simulink model "AariaJoystickR2017a"  (R2017a)
settings: Solver=VariableStepAuto  StartTime=0.0  StopTime=inf  FixedStep=0.1  RelTol=1e-3  EnableMultiTasking=on
model workspace (MATLAB code in the model file):
  | my_a =1;
undefined symbols (not defined in the file or in its folder): AARIAENV, AARIAMAN, AARIASEN, Camera, sensor, Source_TS, X, Y, Z
libraries: sm_lib x723, nesl_utility x640, dspmathops x314, simulink x168, vrlib x2, powerlib_meascontrol x1, aerolibanimutils x1, aerolibutil x1
(part 16 of 26)

== system AariaJoystickR2017a/Joint2/JointVSS/PrismaticTorque/IMU Sensors/Sensor Module1 ==
  Gain : Gain  Gain=1/AARIAENV.Min_TS
  Gain1 : Gain  Gain=1/AARIAENV.Min_TS^2
  Gain3 : Gain  Gain=AARIAENV.gravity  Multiplication=Matrix(K*u)
  Mux : Mux  Inputs=3
  Mux1 : Mux  Inputs=3
  Mux2 : Mux  Inputs=3
  PS-Simulink Converter{5..11} (7 alike) : nesl_utility/PS-Simulink Converter  PhysicalDomain=network_engine_domain  SubClassName=ps_output  LeftPortType=input  RightPortType=output  PseudoPeriodic=off  Frequencies=[]  Unit=1  AffineConversion=off
  PS-Simulink Converter2 : nesl_utility/PS-Simulink Converter  PhysicalDomain=network_engine_domain  SubClassName=ps_output  LeftPortType=input  RightPortType=output  PseudoPeriodic=off  Frequencies=[]  Unit=rad/s  AffineConversion=off
  PS-Simulink Converter3 : nesl_utility/PS-Simulink Converter  PhysicalDomain=network_engine_domain  SubClassName=ps_output  LeftPortType=input  RightPortType=output  PseudoPeriodic=off  Frequencies=[]  Unit=rad/s  AffineConversion=off
  PS-Simulink Converter4 : nesl_utility/PS-Simulink Converter  PhysicalDomain=network_engine_domain  SubClassName=ps_output  LeftPortType=input  RightPortType=output  PseudoPeriodic=off  Frequencies=[]  Unit=rad/s  AffineConversion=off
  Sensor Place : sm_lib/Frames and Transforms/Rigid Transform  TranslationMethod=Cartesian  TranslationStandardOffset=0  TranslationLengthUnit=m  TranslationStandardAxis=+Z  TranslationCartesianOffset=AARIAMAN.L(nL).S(nS).pose_p  TranslationROffset=0  TranslationROffsetUnits=m  TranslationZOffset=0  TranslationZOffsetUnits=m  TranslationThetaOffset=0  TranslationThetaOffsetUnits=deg  RotationMethod=RotationMatrix  RotationAngleUnits=deg  RotationStandardAxis=+Z  RotationAngle=0.0  RotationArbitraryAxis=[0 0 1]  FollAlignAxisA=+X  BaseAlignAxisA=+Y  FollAlignAxisB=+Y  BaseAlignAxisB=+Z  RotationSequenceAxes=FollowerAxes  RotationSequence=XYX  RotationSequenceAngles=[0 0 0]  RotationSequenceAnglesUnits=deg  RotationMatrix=AARIAMAN.L(nL).S(nS).pose_r
  Sum : Sum  Inputs=|++
  Sum1 : Sum  Inputs=|++
  Sum2 : Sum  Inputs=++|
  Transform Sensor : sm_lib/Frames and Transforms/Transform Sensor  MeasurementFrame=Follower  SenseAngle=off  SenseAxis=off  SenseAngle1=off  SenseAngle2=off  SenseAngle3=off  SenseQ=off  SenseR=on  SenseOmegaX=on  SenseOmegaY=on  SenseOmegaZ=on  SenseOmega1=off  SenseOmega2=off  SenseOmega3=off  SenseQDot=off  SenseRDot=off  SenseAlphaX=off  SenseAlphaY=off  SenseAlphaZ=off  SenseAlpha1=off  SenseAlpha2=off  SenseAlpha3=off  SenseQDDot=off  SenseRDDot=off  SenseX=on  SenseY=on  SenseZ=on  SenseRad=off  SenseAzim=off  SenseDist=off  SenseInc=off  SenseXDot=off  SenseYDot=off  SenseZDot=off  SenseRadDot=off  SenseAzimDot=off  SenseDistDot=off  SenseIncDot=off  SenseXDDot=on  SenseYDDot=on  SenseZDDot=on  SenseRadDDot=off  SenseAzimDDot=off  SenseDistDDot=off  SenseIncDDot=off
  a_noise : Subsystem
  coord_sens : sm_lib/Body Elements/Graphic  GraphicType=Marker  MarkerShape=Frame  MarkerSize=AARIAMAN.vis.coord_sizeS  GraphicVisPropType=SimpleVisualProperties  GraphicDiffuseColor=AARIAMAN.vis.col_s  GraphicSpecularColor=[0.5 0.5 0.5 1.0]  GraphicAmbientColor=[0.15 0.15 0.15 1.0]  GraphicEmissiveColor=[0.0 0.0 0.0 1.0]  GraphicShininess=75  GraphicOpacity=AARIAMAN.vis.opacity_s
      settings: SourceProductName=Simscape Multibody
  omega_noise : Subsystem
  Body Frame : PMIOPort  Port=1  Side=Left
  Reference Frame : PMIOPort  Port=2  Side=Left
  Out5 : Outport
  Out4 : Outport  Port=2
  Out2 : Outport  Port=3
  Out3 : Outport  Port=4
  wires:
  Gain1/1 -> Sum/1
  Gain/1 -> Sum2/2
  a_noise/1(noise) -> Sum1/2
  omega_noise/1(noise) -> Sum2/1
  Gain3/1 -> Sum/2  "a_measured"
  Sum1/1 -> Out4/1  "a_measured"
  PS-Simulink Converter10/1 -> Mux2/2
  Mux1/1 -> Out2/1  "P_actual"
  PS-Simulink Converter11/1 -> Mux2/3
  PS-Simulink Converter9/1 -> Mux2/1
  PS-Simulink Converter3/1 -> Mux/2
  PS-Simulink Converter2/1 -> Mux/1
  PS-Simulink Converter4/1 -> Mux/3
  Mux/1 -> Gain/1
  PS-Simulink Converter6/1 -> Mux1/2
  PS-Simulink Converter5/1 -> Mux1/1
  PS-Simulink Converter7/1 -> Mux1/3
  Mux2/1 -> Gain1/1
  PS-Simulink Converter8/1 -> Out3/1, Gain3/1  "R_actual"
  Sum/1 -> Sum1/1
  Sum2/1 -> Out5/1  "omega_measured"
  connections:
  Sensor Place/RConn1 -- coord_sens/RConn1 -- Transform Sensor/RConn1
  Transform Sensor/RConn11 -- PS-Simulink Converter11/LConn1
  Sensor Place/LConn1 -- Body Frame/RConn1
  Transform Sensor/RConn3 -- PS-Simulink Converter2/LConn1
  Transform Sensor/RConn9 -- PS-Simulink Converter9/LConn1
  Transform Sensor/RConn4 -- PS-Simulink Converter3/LConn1
  Transform Sensor/LConn1 -- Reference Frame/RConn1
  Transform Sensor/RConn5 -- PS-Simulink Converter4/LConn1
  Transform Sensor/RConn10 -- PS-Simulink Converter10/LConn1
  Transform Sensor/RConn6 -- PS-Simulink Converter5/LConn1
  PS-Simulink Converter8/LConn1 -- Transform Sensor/RConn2
  Transform Sensor/RConn8 -- PS-Simulink Converter7/LConn1
  Transform Sensor/RConn7 -- PS-Simulink Converter6/LConn1

== system AariaJoystickR2017a/Joint2/JointVSS/PrismaticTorque/IMU Sensors/Sensor Module2 ==
  Gain : Gain  Gain=1/AARIAENV.Min_TS
  Gain1 : Gain  Gain=1/AARIAENV.Min_TS^2
  Gain3 : Gain  Gain=AARIAENV.gravity  Multiplication=Matrix(K*u)
  Mux : Mux  Inputs=3
  Mux1 : Mux  Inputs=3
  Mux2 : Mux  Inputs=3
  PS-Simulink Converter{5..11} (7 alike) : nesl_utility/PS-Simulink Converter  PhysicalDomain=network_engine_domain  SubClassName=ps_output  LeftPortType=input  RightPortType=output  PseudoPeriodic=off  Frequencies=[]  Unit=1  AffineConversion=off
  PS-Simulink Converter2 : nesl_utility/PS-Simulink Converter  PhysicalDomain=network_engine_domain  SubClassName=ps_output  LeftPortType=input  RightPortType=output  PseudoPeriodic=off  Frequencies=[]  Unit=rad/s  AffineConversion=off
  PS-Simulink Converter3 : nesl_utility/PS-Simulink Converter  PhysicalDomain=network_engine_domain  SubClassName=ps_output  LeftPortType=input  RightPortType=output  PseudoPeriodic=off  Frequencies=[]  Unit=rad/s  AffineConversion=off
  PS-Simulink Converter4 : nesl_utility/PS-Simulink Converter  PhysicalDomain=network_engine_domain  SubClassName=ps_output  LeftPortType=input  RightPortType=output  PseudoPeriodic=off  Frequencies=[]  Unit=rad/s  AffineConversion=off
  Sensor Place : sm_lib/Frames and Transforms/Rigid Transform  TranslationMethod=Cartesian  TranslationStandardOffset=0  TranslationLengthUnit=m  TranslationStandardAxis=+Z  TranslationCartesianOffset=AARIAMAN.L(nL).S(nS).pose_p  TranslationROffset=0  TranslationROffsetUnits=m  TranslationZOffset=0  TranslationZOffsetUnits=m  TranslationThetaOffset=0  TranslationThetaOffsetUnits=deg  RotationMethod=RotationMatrix  RotationAngleUnits=deg  RotationStandardAxis=+Z  RotationAngle=0.0  RotationArbitraryAxis=[0 0 1]  FollAlignAxisA=+X  BaseAlignAxisA=+Y  FollAlignAxisB=+Y  BaseAlignAxisB=+Z  RotationSequenceAxes=FollowerAxes  RotationSequence=XYX  RotationSequenceAngles=[0 0 0]  RotationSequenceAnglesUnits=deg  RotationMatrix=AARIAMAN.L(nL).S(nS).pose_r
  Sum : Sum  Inputs=|++
  Sum1 : Sum  Inputs=|++
  Sum2 : Sum  Inputs=++|
  Transform Sensor : sm_lib/Frames and Transforms/Transform Sensor  MeasurementFrame=Follower  SenseAngle=off  SenseAxis=off  SenseAngle1=off  SenseAngle2=off  SenseAngle3=off  SenseQ=off  SenseR=on  SenseOmegaX=on  SenseOmegaY=on  SenseOmegaZ=on  SenseOmega1=off  SenseOmega2=off  SenseOmega3=off  SenseQDot=off  SenseRDot=off  SenseAlphaX=off  SenseAlphaY=off  SenseAlphaZ=off  SenseAlpha1=off  SenseAlpha2=off  SenseAlpha3=off  SenseQDDot=off  SenseRDDot=off  SenseX=on  SenseY=on  SenseZ=on  SenseRad=off  SenseAzim=off  SenseDist=off  SenseInc=off  SenseXDot=off  SenseYDot=off  SenseZDot=off  SenseRadDot=off  SenseAzimDot=off  SenseDistDot=off  SenseIncDot=off  SenseXDDot=on  SenseYDDot=on  SenseZDDot=on  SenseRadDDot=off  SenseAzimDDot=off  SenseDistDDot=off  SenseIncDDot=off
  a_noise : Subsystem
  coord_sens : sm_lib/Body Elements/Graphic  GraphicType=Marker  MarkerShape=Frame  MarkerSize=AARIAMAN.vis.coord_sizeS  GraphicVisPropType=SimpleVisualProperties  GraphicDiffuseColor=AARIAMAN.vis.col_s  GraphicSpecularColor=[0.5 0.5 0.5 1.0]  GraphicAmbientColor=[0.15 0.15 0.15 1.0]  GraphicEmissiveColor=[0.0 0.0 0.0 1.0]  GraphicShininess=75  GraphicOpacity=AARIAMAN.vis.opacity_s
      settings: SourceProductName=Simscape Multibody
  omega_noise : Subsystem
  Body Frame : PMIOPort  Port=1  Side=Left
  Reference Frame : PMIOPort  Port=2  Side=Left
  Out5 : Outport
  Out4 : Outport  Port=2
  Out2 : Outport  Port=3
  Out3 : Outport  Port=4
  wires:
  Gain1/1 -> Sum/1
  Gain/1 -> Sum2/2
  a_noise/1(noise) -> Sum1/2
  omega_noise/1(noise) -> Sum2/1
  Gain3/1 -> Sum/2  "a_measured"
  Sum1/1 -> Out4/1  "a_measured"
  PS-Simulink Converter10/1 -> Mux2/2
  Mux1/1 -> Out2/1  "P_actual"
  PS-Simulink Converter11/1 -> Mux2/3
  PS-Simulink Converter9/1 -> Mux2/1
  PS-Simulink Converter3/1 -> Mux/2
  PS-Simulink Converter2/1 -> Mux/1
  PS-Simulink Converter4/1 -> Mux/3
  Mux/1 -> Gain/1
  PS-Simulink Converter6/1 -> Mux1/2
  PS-Simulink Converter5/1 -> Mux1/1
  PS-Simulink Converter7/1 -> Mux1/3
  Mux2/1 -> Gain1/1
  PS-Simulink Converter8/1 -> Out3/1, Gain3/1  "R_actual"
  Sum/1 -> Sum1/1
  Sum2/1 -> Out5/1  "omega_measured"
  connections:
  Sensor Place/RConn1 -- coord_sens/RConn1 -- Transform Sensor/RConn1
  Transform Sensor/RConn11 -- PS-Simulink Converter11/LConn1
  Sensor Place/LConn1 -- Body Frame/RConn1
  Transform Sensor/RConn3 -- PS-Simulink Converter2/LConn1
  Transform Sensor/RConn9 -- PS-Simulink Converter9/LConn1
  Transform Sensor/RConn4 -- PS-Simulink Converter3/LConn1
  Transform Sensor/LConn1 -- Reference Frame/RConn1
  Transform Sensor/RConn5 -- PS-Simulink Converter4/LConn1
  Transform Sensor/RConn10 -- PS-Simulink Converter10/LConn1
  Transform Sensor/RConn6 -- PS-Simulink Converter5/LConn1
  PS-Simulink Converter8/LConn1 -- Transform Sensor/RConn2
  Transform Sensor/RConn8 -- PS-Simulink Converter7/LConn1
  Transform Sensor/RConn7 -- PS-Simulink Converter6/LConn1

== system AariaJoystickR2017a/Joint2/JointVSS/RevoluteMotion/IMU Sensors/Sensor Module1 ==
  Gain : Gain  Gain=1/AARIAENV.Min_TS
  Gain1 : Gain  Gain=1/AARIAENV.Min_TS^2
  Gain3 : Gain  Gain=AARIAENV.gravity  Multiplication=Matrix(K*u)
  Mux : Mux  Inputs=3
  Mux1 : Mux  Inputs=3
  Mux2 : Mux  Inputs=3
  PS-Simulink Converter{5..11} (7 alike) : nesl_utility/PS-Simulink Converter  PhysicalDomain=network_engine_domain  SubClassName=ps_output  LeftPortType=input  RightPortType=output  PseudoPeriodic=off  Frequencies=[]  Unit=1  AffineConversion=off
  PS-Simulink Converter2 : nesl_utility/PS-Simulink Converter  PhysicalDomain=network_engine_domain  SubClassName=ps_output  LeftPortType=input  RightPortType=output  PseudoPeriodic=off  Frequencies=[]  Unit=rad/s  AffineConversion=off
  PS-Simulink Converter3 : nesl_utility/PS-Simulink Converter  PhysicalDomain=network_engine_domain  SubClassName=ps_output  LeftPortType=input  RightPortType=output  PseudoPeriodic=off  Frequencies=[]  Unit=rad/s  AffineConversion=off
  PS-Simulink Converter4 : nesl_utility/PS-Simulink Converter  PhysicalDomain=network_engine_domain  SubClassName=ps_output  LeftPortType=input  RightPortType=output  PseudoPeriodic=off  Frequencies=[]  Unit=rad/s  AffineConversion=off
  Sensor Place : sm_lib/Frames and Transforms/Rigid Transform  TranslationMethod=Cartesian  TranslationStandardOffset=0  TranslationLengthUnit=m  TranslationStandardAxis=+Z  TranslationCartesianOffset=AARIAMAN.L(nL).S(nS).pose_p  TranslationROffset=0  TranslationROffsetUnits=m  TranslationZOffset=0  TranslationZOffsetUnits=m  TranslationThetaOffset=0  TranslationThetaOffsetUnits=deg  RotationMethod=RotationMatrix  RotationAngleUnits=deg  RotationStandardAxis=+Z  RotationAngle=0.0  RotationArbitraryAxis=[0 0 1]  FollAlignAxisA=+X  BaseAlignAxisA=+Y  FollAlignAxisB=+Y  BaseAlignAxisB=+Z  RotationSequenceAxes=FollowerAxes  RotationSequence=XYX  RotationSequenceAngles=[0 0 0]  RotationSequenceAnglesUnits=deg  RotationMatrix=AARIAMAN.L(nL).S(nS).pose_r
  Sum : Sum  Inputs=|++
  Sum1 : Sum  Inputs=|++
  Sum2 : Sum  Inputs=++|
  Transform Sensor : sm_lib/Frames and Transforms/Transform Sensor  MeasurementFrame=Follower  SenseAngle=off  SenseAxis=off  SenseAngle1=off  SenseAngle2=off  SenseAngle3=off  SenseQ=off  SenseR=on  SenseOmegaX=on  SenseOmegaY=on  SenseOmegaZ=on  SenseOmega1=off  SenseOmega2=off  SenseOmega3=off  SenseQDot=off  SenseRDot=off  SenseAlphaX=off  SenseAlphaY=off  SenseAlphaZ=off  SenseAlpha1=off  SenseAlpha2=off  SenseAlpha3=off  SenseQDDot=off  SenseRDDot=off  SenseX=on  SenseY=on  SenseZ=on  SenseRad=off  SenseAzim=off  SenseDist=off  SenseInc=off  SenseXDot=off  SenseYDot=off  SenseZDot=off  SenseRadDot=off  SenseAzimDot=off  SenseDistDot=off  SenseIncDot=off  SenseXDDot=on  SenseYDDot=on  SenseZDDot=on  SenseRadDDot=off  SenseAzimDDot=off  SenseDistDDot=off  SenseIncDDot=off
  a_noise : Subsystem
  coord_sens : sm_lib/Body Elements/Graphic  GraphicType=Marker  MarkerShape=Frame  MarkerSize=AARIAMAN.vis.coord_sizeS  GraphicVisPropType=SimpleVisualProperties  GraphicDiffuseColor=AARIAMAN.vis.col_s  GraphicSpecularColor=[0.5 0.5 0.5 1.0]  GraphicAmbientColor=[0.15 0.15 0.15 1.0]  GraphicEmissiveColor=[0.0 0.0 0.0 1.0]  GraphicShininess=75  GraphicOpacity=AARIAMAN.vis.opacity_s
      settings: SourceProductName=Simscape Multibody
  omega_noise : Subsystem
  Body Frame : PMIOPort  Port=1  Side=Left
  Reference Frame : PMIOPort  Port=2  Side=Left
  Out5 : Outport
  Out4 : Outport  Port=2
  Out2 : Outport  Port=3
  Out3 : Outport  Port=4
  wires:
  Gain1/1 -> Sum/1
  Gain/1 -> Sum2/2
  a_noise/1(noise) -> Sum1/2
  omega_noise/1(noise) -> Sum2/1
  Gain3/1 -> Sum/2  "a_measured"
  Sum1/1 -> Out4/1  "a_measured"
  PS-Simulink Converter10/1 -> Mux2/2
  Mux1/1 -> Out2/1  "P_actual"
  PS-Simulink Converter11/1 -> Mux2/3
  PS-Simulink Converter9/1 -> Mux2/1
  PS-Simulink Converter3/1 -> Mux/2
  PS-Simulink Converter2/1 -> Mux/1
  PS-Simulink Converter4/1 -> Mux/3
  Mux/1 -> Gain/1
  PS-Simulink Converter6/1 -> Mux1/2
  PS-Simulink Converter5/1 -> Mux1/1
  PS-Simulink Converter7/1 -> Mux1/3
  Mux2/1 -> Gain1/1
  PS-Simulink Converter8/1 -> Out3/1, Gain3/1  "R_actual"
  Sum/1 -> Sum1/1
  Sum2/1 -> Out5/1  "omega_measured"
  connections:
  Sensor Place/RConn1 -- coord_sens/RConn1 -- Transform Sensor/RConn1
  Transform Sensor/RConn11 -- PS-Simulink Converter11/LConn1
  Sensor Place/LConn1 -- Body Frame/RConn1
  Transform Sensor/RConn3 -- PS-Simulink Converter2/LConn1
  Transform Sensor/RConn9 -- PS-Simulink Converter9/LConn1
  Transform Sensor/RConn4 -- PS-Simulink Converter3/LConn1
  Transform Sensor/LConn1 -- Reference Frame/RConn1
  Transform Sensor/RConn5 -- PS-Simulink Converter4/LConn1
  Transform Sensor/RConn10 -- PS-Simulink Converter10/LConn1
  Transform Sensor/RConn6 -- PS-Simulink Converter5/LConn1
  PS-Simulink Converter8/LConn1 -- Transform Sensor/RConn2
  Transform Sensor/RConn8 -- PS-Simulink Converter7/LConn1
  Transform Sensor/RConn7 -- PS-Simulink Converter6/LConn1

== system AariaJoystickR2017a/Joint2/JointVSS/RevoluteMotion/IMU Sensors/Sensor Module2 ==
  Gain : Gain  Gain=1/AARIAENV.Min_TS
  Gain1 : Gain  Gain=1/AARIAENV.Min_TS^2
  Gain3 : Gain  Gain=AARIAENV.gravity  Multiplication=Matrix(K*u)
  Mux : Mux  Inputs=3
  Mux1 : Mux  Inputs=3
  Mux2 : Mux  Inputs=3
  PS-Simulink Converter{5..11} (7 alike) : nesl_utility/PS-Simulink Converter  PhysicalDomain=network_engine_domain  SubClassName=ps_output  LeftPortType=input  RightPortType=output  PseudoPeriodic=off  Frequencies=[]  Unit=1  AffineConversion=off
  PS-Simulink Converter2 : nesl_utility/PS-Simulink Converter  PhysicalDomain=network_engine_domain  SubClassName=ps_output  LeftPortType=input  RightPortType=output  PseudoPeriodic=off  Frequencies=[]  Unit=rad/s  AffineConversion=off
  PS-Simulink Converter3 : nesl_utility/PS-Simulink Converter  PhysicalDomain=network_engine_domain  SubClassName=ps_output  LeftPortType=input  RightPortType=output  PseudoPeriodic=off  Frequencies=[]  Unit=rad/s  AffineConversion=off
  PS-Simulink Converter4 : nesl_utility/PS-Simulink Converter  PhysicalDomain=network_engine_domain  SubClassName=ps_output  LeftPortType=input  RightPortType=output  PseudoPeriodic=off  Frequencies=[]  Unit=rad/s  AffineConversion=off
  Sensor Place : sm_lib/Frames and Transforms/Rigid Transform  TranslationMethod=Cartesian  TranslationStandardOffset=0  TranslationLengthUnit=m  TranslationStandardAxis=+Z  TranslationCartesianOffset=AARIAMAN.L(nL).S(nS).pose_p  TranslationROffset=0  TranslationROffsetUnits=m  TranslationZOffset=0  TranslationZOffsetUnits=m  TranslationThetaOffset=0  TranslationThetaOffsetUnits=deg  RotationMethod=RotationMatrix  RotationAngleUnits=deg  RotationStandardAxis=+Z  RotationAngle=0.0  RotationArbitraryAxis=[0 0 1]  FollAlignAxisA=+X  BaseAlignAxisA=+Y  FollAlignAxisB=+Y  BaseAlignAxisB=+Z  RotationSequenceAxes=FollowerAxes  RotationSequence=XYX  RotationSequenceAngles=[0 0 0]  RotationSequenceAnglesUnits=deg  RotationMatrix=AARIAMAN.L(nL).S(nS).pose_r
  Sum : Sum  Inputs=|++
  Sum1 : Sum  Inputs=|++
  Sum2 : Sum  Inputs=++|
  Transform Sensor : sm_lib/Frames and Transforms/Transform Sensor  MeasurementFrame=Follower  SenseAngle=off  SenseAxis=off  SenseAngle1=off  SenseAngle2=off  SenseAngle3=off  SenseQ=off  SenseR=on  SenseOmegaX=on  SenseOmegaY=on  SenseOmegaZ=on  SenseOmega1=off  SenseOmega2=off  SenseOmega3=off  SenseQDot=off  SenseRDot=off  SenseAlphaX=off  SenseAlphaY=off  SenseAlphaZ=off  SenseAlpha1=off  SenseAlpha2=off  SenseAlpha3=off  SenseQDDot=off  SenseRDDot=off  SenseX=on  SenseY=on  SenseZ=on  SenseRad=off  SenseAzim=off  SenseDist=off  SenseInc=off  SenseXDot=off  SenseYDot=off  SenseZDot=off  SenseRadDot=off  SenseAzimDot=off  SenseDistDot=off  SenseIncDot=off  SenseXDDot=on  SenseYDDot=on  SenseZDDot=on  SenseRadDDot=off  SenseAzimDDot=off  SenseDistDDot=off  SenseIncDDot=off
  a_noise : Subsystem
  coord_sens : sm_lib/Body Elements/Graphic  GraphicType=Marker  MarkerShape=Frame  MarkerSize=AARIAMAN.vis.coord_sizeS  GraphicVisPropType=SimpleVisualProperties  GraphicDiffuseColor=AARIAMAN.vis.col_s  GraphicSpecularColor=[0.5 0.5 0.5 1.0]  GraphicAmbientColor=[0.15 0.15 0.15 1.0]  GraphicEmissiveColor=[0.0 0.0 0.0 1.0]  GraphicShininess=75  GraphicOpacity=AARIAMAN.vis.opacity_s
      settings: SourceProductName=Simscape Multibody
  omega_noise : Subsystem
  Body Frame : PMIOPort  Port=1  Side=Left
  Reference Frame : PMIOPort  Port=2  Side=Left
  Out5 : Outport
  Out4 : Outport  Port=2
  Out2 : Outport  Port=3
  Out3 : Outport  Port=4
  wires:
  Gain1/1 -> Sum/1
  Gain/1 -> Sum2/2
  a_noise/1(noise) -> Sum1/2
  omega_noise/1(noise) -> Sum2/1
  Gain3/1 -> Sum/2  "a_measured"
  Sum1/1 -> Out4/1  "a_measured"
  PS-Simulink Converter10/1 -> Mux2/2
  Mux1/1 -> Out2/1  "P_actual"
  PS-Simulink Converter11/1 -> Mux2/3
  PS-Simulink Converter9/1 -> Mux2/1
  PS-Simulink Converter3/1 -> Mux/2
  PS-Simulink Converter2/1 -> Mux/1
  PS-Simulink Converter4/1 -> Mux/3
  Mux/1 -> Gain/1
  PS-Simulink Converter6/1 -> Mux1/2
  PS-Simulink Converter5/1 -> Mux1/1
  PS-Simulink Converter7/1 -> Mux1/3
  Mux2/1 -> Gain1/1
  PS-Simulink Converter8/1 -> Out3/1, Gain3/1  "R_actual"
  Sum/1 -> Sum1/1
  Sum2/1 -> Out5/1  "omega_measured"
  connections:
  Sensor Place/RConn1 -- coord_sens/RConn1 -- Transform Sensor/RConn1
  Transform Sensor/RConn11 -- PS-Simulink Converter11/LConn1
  Sensor Place/LConn1 -- Body Frame/RConn1
  Transform Sensor/RConn3 -- PS-Simulink Converter2/LConn1
  Transform Sensor/RConn9 -- PS-Simulink Converter9/LConn1
  Transform Sensor/RConn4 -- PS-Simulink Converter3/LConn1
  Transform Sensor/LConn1 -- Reference Frame/RConn1
  Transform Sensor/RConn5 -- PS-Simulink Converter4/LConn1
  Transform Sensor/RConn10 -- PS-Simulink Converter10/LConn1
  Transform Sensor/RConn6 -- PS-Simulink Converter5/LConn1
  PS-Simulink Converter8/LConn1 -- Transform Sensor/RConn2
  Transform Sensor/RConn8 -- PS-Simulink Converter7/LConn1
  Transform Sensor/RConn7 -- PS-Simulink Converter6/LConn1

== system AariaJoystickR2017a/Joint2/JointVSS/RevoluteTorque/IMU Sensors/Sensor Module1 ==
  Gain : Gain  Gain=1/AARIAENV.Min_TS
  Gain1 : Gain  Gain=1/AARIAENV.Min_TS^2
  Gain3 : Gain  Gain=AARIAENV.gravity  Multiplication=Matrix(K*u)
  Mux : Mux  Inputs=3
  Mux1 : Mux  Inputs=3
  Mux2 : Mux  Inputs=3
  PS-Simulink Converter{5..11} (7 alike) : nesl_utility/PS-Simulink Converter  PhysicalDomain=network_engine_domain  SubClassName=ps_output  LeftPortType=input  RightPortType=output  PseudoPeriodic=off  Frequencies=[]  Unit=1  AffineConversion=off
  PS-Simulink Converter2 : nesl_utility/PS-Simulink Converter  PhysicalDomain=network_engine_domain  SubClassName=ps_output  LeftPortType=input  RightPortType=output  PseudoPeriodic=off  Frequencies=[]  Unit=rad/s  AffineConversion=off
  PS-Simulink Converter3 : nesl_utility/PS-Simulink Converter  PhysicalDomain=network_engine_domain  SubClassName=ps_output  LeftPortType=input  RightPortType=output  PseudoPeriodic=off  Frequencies=[]  Unit=rad/s  AffineConversion=off
  PS-Simulink Converter4 : nesl_utility/PS-Simulink Converter  PhysicalDomain=network_engine_domain  SubClassName=ps_output  LeftPortType=input  RightPortType=output  PseudoPeriodic=off  Frequencies=[]  Unit=rad/s  AffineConversion=off
  Sensor Place : sm_lib/Frames and Transforms/Rigid Transform  TranslationMethod=Cartesian  TranslationStandardOffset=0  TranslationLengthUnit=m  TranslationStandardAxis=+Z  TranslationCartesianOffset=AARIAMAN.L(nL).S(nS).pose_p  TranslationROffset=0  TranslationROffsetUnits=m  TranslationZOffset=0  TranslationZOffsetUnits=m  TranslationThetaOffset=0  TranslationThetaOffsetUnits=deg  RotationMethod=RotationMatrix  RotationAngleUnits=deg  RotationStandardAxis=+Z  RotationAngle=0.0  RotationArbitraryAxis=[0 0 1]  FollAlignAxisA=+X  BaseAlignAxisA=+Y  FollAlignAxisB=+Y  BaseAlignAxisB=+Z  RotationSequenceAxes=FollowerAxes  RotationSequence=XYX  RotationSequenceAngles=[0 0 0]  RotationSequenceAnglesUnits=deg  RotationMatrix=AARIAMAN.L(nL).S(nS).pose_r
  Sum : Sum  Inputs=|++
  Sum1 : Sum  Inputs=|++
  Sum2 : Sum  Inputs=++|
  Transform Sensor : sm_lib/Frames and Transforms/Transform Sensor  MeasurementFrame=Follower  SenseAngle=off  SenseAxis=off  SenseAngle1=off  SenseAngle2=off  SenseAngle3=off  SenseQ=off  SenseR=on  SenseOmegaX=on  SenseOmegaY=on  SenseOmegaZ=on  SenseOmega1=off  SenseOmega2=off  SenseOmega3=off  SenseQDot=off  SenseRDot=off  SenseAlphaX=off  SenseAlphaY=off  SenseAlphaZ=off  SenseAlpha1=off  SenseAlpha2=off  SenseAlpha3=off  SenseQDDot=off  SenseRDDot=off  SenseX=on  SenseY=on  SenseZ=on  SenseRad=off  SenseAzim=off  SenseDist=off  SenseInc=off  SenseXDot=off  SenseYDot=off  SenseZDot=off  SenseRadDot=off  SenseAzimDot=off  SenseDistDot=off  SenseIncDot=off  SenseXDDot=on  SenseYDDot=on  SenseZDDot=on  SenseRadDDot=off  SenseAzimDDot=off  SenseDistDDot=off  SenseIncDDot=off
  a_noise : Subsystem
  coord_sens : sm_lib/Body Elements/Graphic  GraphicType=Marker  MarkerShape=Frame  MarkerSize=AARIAMAN.vis.coord_sizeS  GraphicVisPropType=SimpleVisualProperties  GraphicDiffuseColor=AARIAMAN.vis.col_s  GraphicSpecularColor=[0.5 0.5 0.5 1.0]  GraphicAmbientColor=[0.15 0.15 0.15 1.0]  GraphicEmissiveColor=[0.0 0.0 0.0 1.0]  GraphicShininess=75  GraphicOpacity=AARIAMAN.vis.opacity_s
      settings: SourceProductName=Simscape Multibody
  omega_noise : Subsystem
  Body Frame : PMIOPort  Port=1  Side=Left
  Reference Frame : PMIOPort  Port=2  Side=Left
  Out5 : Outport
  Out4 : Outport  Port=2
  Out2 : Outport  Port=3
  Out3 : Outport  Port=4
  wires:
  Gain1/1 -> Sum/1
  Gain/1 -> Sum2/2
  a_noise/1(noise) -> Sum1/2
  omega_noise/1(noise) -> Sum2/1
  Gain3/1 -> Sum/2  "a_measured"
  Sum1/1 -> Out4/1  "a_measured"
  PS-Simulink Converter10/1 -> Mux2/2
  Mux1/1 -> Out2/1  "P_actual"
  PS-Simulink Converter11/1 -> Mux2/3
  PS-Simulink Converter9/1 -> Mux2/1
  PS-Simulink Converter3/1 -> Mux/2
  PS-Simulink Converter2/1 -> Mux/1
  PS-Simulink Converter4/1 -> Mux/3
  Mux/1 -> Gain/1
  PS-Simulink Converter6/1 -> Mux1/2
  PS-Simulink Converter5/1 -> Mux1/1
  PS-Simulink Converter7/1 -> Mux1/3
  Mux2/1 -> Gain1/1
  PS-Simulink Converter8/1 -> Out3/1, Gain3/1  "R_actual"
  Sum/1 -> Sum1/1
  Sum2/1 -> Out5/1  "omega_measured"
  connections:
  Sensor Place/RConn1 -- coord_sens/RConn1 -- Transform Sensor/RConn1
  Transform Sensor/RConn11 -- PS-Simulink Converter11/LConn1
  Sensor Place/LConn1 -- Body Frame/RConn1
  Transform Sensor/RConn3 -- PS-Simulink Converter2/LConn1
  Transform Sensor/RConn9 -- PS-Simulink Converter9/LConn1
  Transform Sensor/RConn4 -- PS-Simulink Converter3/LConn1
  Transform Sensor/LConn1 -- Reference Frame/RConn1
  Transform Sensor/RConn5 -- PS-Simulink Converter4/LConn1
  Transform Sensor/RConn10 -- PS-Simulink Converter10/LConn1
  Transform Sensor/RConn6 -- PS-Simulink Converter5/LConn1
  PS-Simulink Converter8/LConn1 -- Transform Sensor/RConn2
  Transform Sensor/RConn8 -- PS-Simulink Converter7/LConn1
  Transform Sensor/RConn7 -- PS-Simulink Converter6/LConn1

== system AariaJoystickR2017a/Joint2/JointVSS/RevoluteTorque/IMU Sensors/Sensor Module2 ==
  Gain : Gain  Gain=1/AARIAENV.Min_TS
  Gain1 : Gain  Gain=1/AARIAENV.Min_TS^2
  Gain3 : Gain  Gain=AARIAENV.gravity  Multiplication=Matrix(K*u)
  Mux : Mux  Inputs=3
  Mux1 : Mux  Inputs=3
  Mux2 : Mux  Inputs=3
  PS-Simulink Converter{5..11} (7 alike) : nesl_utility/PS-Simulink Converter  PhysicalDomain=network_engine_domain  SubClassName=ps_output  LeftPortType=input  RightPortType=output  PseudoPeriodic=off  Frequencies=[]  Unit=1  AffineConversion=off
  PS-Simulink Converter2 : nesl_utility/PS-Simulink Converter  PhysicalDomain=network_engine_domain  SubClassName=ps_output  LeftPortType=input  RightPortType=output  PseudoPeriodic=off  Frequencies=[]  Unit=rad/s  AffineConversion=off
  PS-Simulink Converter3 : nesl_utility/PS-Simulink Converter  PhysicalDomain=network_engine_domain  SubClassName=ps_output  LeftPortType=input  RightPortType=output  PseudoPeriodic=off  Frequencies=[]  Unit=rad/s  AffineConversion=off
  PS-Simulink Converter4 : nesl_utility/PS-Simulink Converter  PhysicalDomain=network_engine_domain  SubClassName=ps_output  LeftPortType=input  RightPortType=output  PseudoPeriodic=off  Frequencies=[]  Unit=rad/s  AffineConversion=off
  Sensor Place : sm_lib/Frames and Transforms/Rigid Transform  TranslationMethod=Cartesian  TranslationStandardOffset=0  TranslationLengthUnit=m  TranslationStandardAxis=+Z  TranslationCartesianOffset=AARIAMAN.L(nL).S(nS).pose_p  TranslationROffset=0  TranslationROffsetUnits=m  TranslationZOffset=0  TranslationZOffsetUnits=m  TranslationThetaOffset=0  TranslationThetaOffsetUnits=deg  RotationMethod=RotationMatrix  RotationAngleUnits=deg  RotationStandardAxis=+Z  RotationAngle=0.0  RotationArbitraryAxis=[0 0 1]  FollAlignAxisA=+X  BaseAlignAxisA=+Y  FollAlignAxisB=+Y  BaseAlignAxisB=+Z  RotationSequenceAxes=FollowerAxes  RotationSequence=XYX  RotationSequenceAngles=[0 0 0]  RotationSequenceAnglesUnits=deg  RotationMatrix=AARIAMAN.L(nL).S(nS).pose_r
  Sum : Sum  Inputs=|++
  Sum1 : Sum  Inputs=|++
  Sum2 : Sum  Inputs=++|
  Transform Sensor : sm_lib/Frames and Transforms/Transform Sensor  MeasurementFrame=Follower  SenseAngle=off  SenseAxis=off  SenseAngle1=off  SenseAngle2=off  SenseAngle3=off  SenseQ=off  SenseR=on  SenseOmegaX=on  SenseOmegaY=on  SenseOmegaZ=on  SenseOmega1=off  SenseOmega2=off  SenseOmega3=off  SenseQDot=off  SenseRDot=off  SenseAlphaX=off  SenseAlphaY=off  SenseAlphaZ=off  SenseAlpha1=off  SenseAlpha2=off  SenseAlpha3=off  SenseQDDot=off  SenseRDDot=off  SenseX=on  SenseY=on  SenseZ=on  SenseRad=off  SenseAzim=off  SenseDist=off  SenseInc=off  SenseXDot=off  SenseYDot=off  SenseZDot=off  SenseRadDot=off  SenseAzimDot=off  SenseDistDot=off  SenseIncDot=off  SenseXDDot=on  SenseYDDot=on  SenseZDDot=on  SenseRadDDot=off  SenseAzimDDot=off  SenseDistDDot=off  SenseIncDDot=off
  a_noise : Subsystem
  coord_sens : sm_lib/Body Elements/Graphic  GraphicType=Marker  MarkerShape=Frame  MarkerSize=AARIAMAN.vis.coord_sizeS  GraphicVisPropType=SimpleVisualProperties  GraphicDiffuseColor=AARIAMAN.vis.col_s  GraphicSpecularColor=[0.5 0.5 0.5 1.0]  GraphicAmbientColor=[0.15 0.15 0.15 1.0]  GraphicEmissiveColor=[0.0 0.0 0.0 1.0]  GraphicShininess=75  GraphicOpacity=AARIAMAN.vis.opacity_s
      settings: SourceProductName=Simscape Multibody
  omega_noise : Subsystem
  Body Frame : PMIOPort  Port=1  Side=Left
  Reference Frame : PMIOPort  Port=2  Side=Left
  Out5 : Outport
  Out4 : Outport  Port=2
  Out2 : Outport  Port=3
  Out3 : Outport  Port=4
  wires:
  Gain1/1 -> Sum/1
  Gain/1 -> Sum2/2
  a_noise/1(noise) -> Sum1/2
  omega_noise/1(noise) -> Sum2/1
  Gain3/1 -> Sum/2  "a_measured"
  Sum1/1 -> Out4/1  "a_measured"
  PS-Simulink Converter10/1 -> Mux2/2
  Mux1/1 -> Out2/1  "P_actual"
  PS-Simulink Converter11/1 -> Mux2/3
  PS-Simulink Converter9/1 -> Mux2/1
  PS-Simulink Converter3/1 -> Mux/2
  PS-Simulink Converter2/1 -> Mux/1
  PS-Simulink Converter4/1 -> Mux/3
  Mux/1 -> Gain/1
  PS-Simulink Converter6/1 -> Mux1/2
  PS-Simulink Converter5/1 -> Mux1/1
  PS-Simulink Converter7/1 -> Mux1/3
  Mux2/1 -> Gain1/1
  PS-Simulink Converter8/1 -> Out3/1, Gain3/1  "R_actual"
  Sum/1 -> Sum1/1
  Sum2/1 -> Out5/1  "omega_measured"
  connections:
  Sensor Place/RConn1 -- coord_sens/RConn1 -- Transform Sensor/RConn1
  Transform Sensor/RConn11 -- PS-Simulink Converter11/LConn1
  Sensor Place/LConn1 -- Body Frame/RConn1
  Transform Sensor/RConn3 -- PS-Simulink Converter2/LConn1
  Transform Sensor/RConn9 -- PS-Simulink Converter9/LConn1
  Transform Sensor/RConn4 -- PS-Simulink Converter3/LConn1
  Transform Sensor/LConn1 -- Reference Frame/RConn1
  Transform Sensor/RConn5 -- PS-Simulink Converter4/LConn1
  Transform Sensor/RConn10 -- PS-Simulink Converter10/LConn1
  Transform Sensor/RConn6 -- PS-Simulink Converter5/LConn1
  PS-Simulink Converter8/LConn1 -- Transform Sensor/RConn2
  Transform Sensor/RConn8 -- PS-Simulink Converter7/LConn1
  Transform Sensor/RConn7 -- PS-Simulink Converter6/LConn1

== system AariaJoystickR2017a/Joint3/JointVSS/PrismaticMotion/IMU Sensors/Sensor Module1 ==
  Gain : Gain  Gain=1/AARIAENV.Min_TS
  Gain1 : Gain  Gain=1/AARIAENV.Min_TS^2
  Gain3 : Gain  Gain=AARIAENV.gravity  Multiplication=Matrix(K*u)
  Mux : Mux  Inputs=3
  Mux1 : Mux  Inputs=3
  Mux2 : Mux  Inputs=3
  PS-Simulink Converter{5..11} (7 alike) : nesl_utility/PS-Simulink Converter  PhysicalDomain=network_engine_domain  SubClassName=ps_output  LeftPortType=input  RightPortType=output  PseudoPeriodic=off  Frequencies=[]  Unit=1  AffineConversion=off
  PS-Simulink Converter2 : nesl_utility/PS-Simulink Converter  PhysicalDomain=network_engine_domain  SubClassName=ps_output  LeftPortType=input  RightPortType=output  PseudoPeriodic=off  Frequencies=[]  Unit=rad/s  AffineConversion=off
  PS-Simulink Converter3 : nesl_utility/PS-Simulink Converter  PhysicalDomain=network_engine_domain  SubClassName=ps_output  LeftPortType=input  RightPortType=output  PseudoPeriodic=off  Frequencies=[]  Unit=rad/s  AffineConversion=off
  PS-Simulink Converter4 : nesl_utility/PS-Simulink Converter  PhysicalDomain=network_engine_domain  SubClassName=ps_output  LeftPortType=input  RightPortType=output  PseudoPeriodic=off  Frequencies=[]  Unit=rad/s  AffineConversion=off
  Sensor Place : sm_lib/Frames and Transforms/Rigid Transform  TranslationMethod=Cartesian  TranslationStandardOffset=0  TranslationLengthUnit=m  TranslationStandardAxis=+Z  TranslationCartesianOffset=AARIAMAN.L(nL).S(nS).pose_p  TranslationROffset=0  TranslationROffsetUnits=m  TranslationZOffset=0  TranslationZOffsetUnits=m  TranslationThetaOffset=0  TranslationThetaOffsetUnits=deg  RotationMethod=RotationMatrix  RotationAngleUnits=deg  RotationStandardAxis=+Z  RotationAngle=0.0  RotationArbitraryAxis=[0 0 1]  FollAlignAxisA=+X  BaseAlignAxisA=+Y  FollAlignAxisB=+Y  BaseAlignAxisB=+Z  RotationSequenceAxes=FollowerAxes  RotationSequence=XYX  RotationSequenceAngles=[0 0 0]  RotationSequenceAnglesUnits=deg  RotationMatrix=AARIAMAN.L(nL).S(nS).pose_r
  Sum : Sum  Inputs=|++
  Sum1 : Sum  Inputs=|++
  Sum2 : Sum  Inputs=++|
  Transform Sensor : sm_lib/Frames and Transforms/Transform Sensor  MeasurementFrame=Follower  SenseAngle=off  SenseAxis=off  SenseAngle1=off  SenseAngle2=off  SenseAngle3=off  SenseQ=off  SenseR=on  SenseOmegaX=on  SenseOmegaY=on  SenseOmegaZ=on  SenseOmega1=off  SenseOmega2=off  SenseOmega3=off  SenseQDot=off  SenseRDot=off  SenseAlphaX=off  SenseAlphaY=off  SenseAlphaZ=off  SenseAlpha1=off  SenseAlpha2=off  SenseAlpha3=off  SenseQDDot=off  SenseRDDot=off  SenseX=on  SenseY=on  SenseZ=on  SenseRad=off  SenseAzim=off  SenseDist=off  SenseInc=off  SenseXDot=off  SenseYDot=off  SenseZDot=off  SenseRadDot=off  SenseAzimDot=off  SenseDistDot=off  SenseIncDot=off  SenseXDDot=on  SenseYDDot=on  SenseZDDot=on  SenseRadDDot=off  SenseAzimDDot=off  SenseDistDDot=off  SenseIncDDot=off
  a_noise : Subsystem
  coord_sens : sm_lib/Body Elements/Graphic  GraphicType=Marker  MarkerShape=Frame  MarkerSize=AARIAMAN.vis.coord_sizeS  GraphicVisPropType=SimpleVisualProperties  GraphicDiffuseColor=AARIAMAN.vis.col_s  GraphicSpecularColor=[0.5 0.5 0.5 1.0]  GraphicAmbientColor=[0.15 0.15 0.15 1.0]  GraphicEmissiveColor=[0.0 0.0 0.0 1.0]  GraphicShininess=75  GraphicOpacity=AARIAMAN.vis.opacity_s
      settings: SourceProductName=Simscape Multibody
  omega_noise : Subsystem
  Body Frame : PMIOPort  Port=1  Side=Left
  Reference Frame : PMIOPort  Port=2  Side=Left
  Out5 : Outport
  Out4 : Outport  Port=2
  Out2 : Outport  Port=3
  Out3 : Outport  Port=4
  wires:
  Sum2/1 -> Out5/1  "omega_measured"
  Sum/1 -> Sum1/1
  PS-Simulink Converter8/1 -> Gain3/1, Out3/1  "R_actual"
  Mux2/1 -> Gain1/1
  PS-Simulink Converter7/1 -> Mux1/3
  PS-Simulink Converter5/1 -> Mux1/1
  PS-Simulink Converter6/1 -> Mux1/2
  Mux/1 -> Gain/1
  PS-Simulink Converter4/1 -> Mux/3
  PS-Simulink Converter2/1 -> Mux/1
  PS-Simulink Converter3/1 -> Mux/2
  PS-Simulink Converter9/1 -> Mux2/1
  PS-Simulink Converter11/1 -> Mux2/3
  Mux1/1 -> Out2/1  "P_actual"
  PS-Simulink Converter10/1 -> Mux2/2
  Sum1/1 -> Out4/1  "a_measured"
  Gain3/1 -> Sum/2  "a_measured"
  omega_noise/1(noise) -> Sum2/1
  a_noise/1(noise) -> Sum1/2
  Gain/1 -> Sum2/2
  Gain1/1 -> Sum/1
  connections:
  Transform Sensor/RConn7 -- PS-Simulink Converter6/LConn1
  Transform Sensor/RConn8 -- PS-Simulink Converter7/LConn1
  PS-Simulink Converter8/LConn1 -- Transform Sensor/RConn2
  Transform Sensor/RConn6 -- PS-Simulink Converter5/LConn1
  Transform Sensor/RConn10 -- PS-Simulink Converter10/LConn1
  Transform Sensor/RConn5 -- PS-Simulink Converter4/LConn1
  Transform Sensor/LConn1 -- Reference Frame/RConn1
  Transform Sensor/RConn4 -- PS-Simulink Converter3/LConn1
  Transform Sensor/RConn9 -- PS-Simulink Converter9/LConn1
  Transform Sensor/RConn3 -- PS-Simulink Converter2/LConn1
  Sensor Place/LConn1 -- Body Frame/RConn1
  Transform Sensor/RConn11 -- PS-Simulink Converter11/LConn1
  Transform Sensor/RConn1 -- coord_sens/RConn1 -- Sensor Place/RConn1

== system AariaJoystickR2017a/Joint3/JointVSS/PrismaticMotion/IMU Sensors/Sensor Module2 ==
  Gain : Gain  Gain=1/AARIAENV.Min_TS
  Gain1 : Gain  Gain=1/AARIAENV.Min_TS^2
  Gain3 : Gain  Gain=AARIAENV.gravity  Multiplication=Matrix(K*u)
  Mux : Mux  Inputs=3
  Mux1 : Mux  Inputs=3
  Mux2 : Mux  Inputs=3
  PS-Simulink Converter{5..11} (7 alike) : nesl_utility/PS-Simulink Converter  PhysicalDomain=network_engine_domain  SubClassName=ps_output  LeftPortType=input  RightPortType=output  PseudoPeriodic=off  Frequencies=[]  Unit=1  AffineConversion=off
  PS-Simulink Converter2 : nesl_utility/PS-Simulink Converter  PhysicalDomain=network_engine_domain  SubClassName=ps_output  LeftPortType=input  RightPortType=output  PseudoPeriodic=off  Frequencies=[]  Unit=rad/s  AffineConversion=off
  PS-Simulink Converter3 : nesl_utility/PS-Simulink Converter  PhysicalDomain=network_engine_domain  SubClassName=ps_output  LeftPortType=input  RightPortType=output  PseudoPeriodic=off  Frequencies=[]  Unit=rad/s  AffineConversion=off
  PS-Simulink Converter4 : nesl_utility/PS-Simulink Converter  PhysicalDomain=network_engine_domain  SubClassName=ps_output  LeftPortType=input  RightPortType=output  PseudoPeriodic=off  Frequencies=[]  Unit=rad/s  AffineConversion=off
  Sensor Place : sm_lib/Frames and Transforms/Rigid Transform  TranslationMethod=Cartesian  TranslationStandardOffset=0  TranslationLengthUnit=m  TranslationStandardAxis=+Z  TranslationCartesianOffset=AARIAMAN.L(nL).S(nS).pose_p  TranslationROffset=0  TranslationROffsetUnits=m  TranslationZOffset=0  TranslationZOffsetUnits=m  TranslationThetaOffset=0  TranslationThetaOffsetUnits=deg  RotationMethod=RotationMatrix  RotationAngleUnits=deg  RotationStandardAxis=+Z  RotationAngle=0.0  RotationArbitraryAxis=[0 0 1]  FollAlignAxisA=+X  BaseAlignAxisA=+Y  FollAlignAxisB=+Y  BaseAlignAxisB=+Z  RotationSequenceAxes=FollowerAxes  RotationSequence=XYX  RotationSequenceAngles=[0 0 0]  RotationSequenceAnglesUnits=deg  RotationMatrix=AARIAMAN.L(nL).S(nS).pose_r
  Sum : Sum  Inputs=|++
  Sum1 : Sum  Inputs=|++
  Sum2 : Sum  Inputs=++|
  Transform Sensor : sm_lib/Frames and Transforms/Transform Sensor  MeasurementFrame=Follower  SenseAngle=off  SenseAxis=off  SenseAngle1=off  SenseAngle2=off  SenseAngle3=off  SenseQ=off  SenseR=on  SenseOmegaX=on  SenseOmegaY=on  SenseOmegaZ=on  SenseOmega1=off  SenseOmega2=off  SenseOmega3=off  SenseQDot=off  SenseRDot=off  SenseAlphaX=off  SenseAlphaY=off  SenseAlphaZ=off  SenseAlpha1=off  SenseAlpha2=off  SenseAlpha3=off  SenseQDDot=off  SenseRDDot=off  SenseX=on  SenseY=on  SenseZ=on  SenseRad=off  SenseAzim=off  SenseDist=off  SenseInc=off  SenseXDot=off  SenseYDot=off  SenseZDot=off  SenseRadDot=off  SenseAzimDot=off  SenseDistDot=off  SenseIncDot=off  SenseXDDot=on  SenseYDDot=on  SenseZDDot=on  SenseRadDDot=off  SenseAzimDDot=off  SenseDistDDot=off  SenseIncDDot=off
  a_noise : Subsystem
  coord_sens : sm_lib/Body Elements/Graphic  GraphicType=Marker  MarkerShape=Frame  MarkerSize=AARIAMAN.vis.coord_sizeS  GraphicVisPropType=SimpleVisualProperties  GraphicDiffuseColor=AARIAMAN.vis.col_s  GraphicSpecularColor=[0.5 0.5 0.5 1.0]  GraphicAmbientColor=[0.15 0.15 0.15 1.0]  GraphicEmissiveColor=[0.0 0.0 0.0 1.0]  GraphicShininess=75  GraphicOpacity=AARIAMAN.vis.opacity_s
      settings: SourceProductName=Simscape Multibody
  omega_noise : Subsystem
  Body Frame : PMIOPort  Port=1  Side=Left
  Reference Frame : PMIOPort  Port=2  Side=Left
  Out5 : Outport
  Out4 : Outport  Port=2
  Out2 : Outport  Port=3
  Out3 : Outport  Port=4
  wires:
  Sum2/1 -> Out5/1  "omega_measured"
  Sum/1 -> Sum1/1
  PS-Simulink Converter8/1 -> Gain3/1, Out3/1  "R_actual"
  Mux2/1 -> Gain1/1
  PS-Simulink Converter7/1 -> Mux1/3
  PS-Simulink Converter5/1 -> Mux1/1
  PS-Simulink Converter6/1 -> Mux1/2
  Mux/1 -> Gain/1
  PS-Simulink Converter4/1 -> Mux/3
  PS-Simulink Converter2/1 -> Mux/1
  PS-Simulink Converter3/1 -> Mux/2
  PS-Simulink Converter9/1 -> Mux2/1
  PS-Simulink Converter11/1 -> Mux2/3
  Mux1/1 -> Out2/1  "P_actual"
  PS-Simulink Converter10/1 -> Mux2/2
  Sum1/1 -> Out4/1  "a_measured"
  Gain3/1 -> Sum/2  "a_measured"
  omega_noise/1(noise) -> Sum2/1
  a_noise/1(noise) -> Sum1/2
  Gain/1 -> Sum2/2
  Gain1/1 -> Sum/1
  connections:
  Transform Sensor/RConn7 -- PS-Simulink Converter6/LConn1
  Transform Sensor/RConn8 -- PS-Simulink Converter7/LConn1
  PS-Simulink Converter8/LConn1 -- Transform Sensor/RConn2
  Transform Sensor/RConn6 -- PS-Simulink Converter5/LConn1
  Transform Sensor/RConn10 -- PS-Simulink Converter10/LConn1
  Transform Sensor/RConn5 -- PS-Simulink Converter4/LConn1
  Transform Sensor/LConn1 -- Reference Frame/RConn1
  Transform Sensor/RConn4 -- PS-Simulink Converter3/LConn1
  Transform Sensor/RConn9 -- PS-Simulink Converter9/LConn1
  Transform Sensor/RConn3 -- PS-Simulink Converter2/LConn1
  Sensor Place/LConn1 -- Body Frame/RConn1
  Transform Sensor/RConn11 -- PS-Simulink Converter11/LConn1
  Transform Sensor/RConn1 -- coord_sens/RConn1 -- Sensor Place/RConn1

== system AariaJoystickR2017a/Joint3/JointVSS/PrismaticTorque/IMU Sensors/Sensor Module1 ==
  Gain : Gain  Gain=1/AARIAENV.Min_TS
  Gain1 : Gain  Gain=1/AARIAENV.Min_TS^2
  Gain3 : Gain  Gain=AARIAENV.gravity  Multiplication=Matrix(K*u)
  Mux : Mux  Inputs=3
  Mux1 : Mux  Inputs=3
  Mux2 : Mux  Inputs=3
  PS-Simulink Converter{5..11} (7 alike) : nesl_utility/PS-Simulink Converter  PhysicalDomain=network_engine_domain  SubClassName=ps_output  LeftPortType=input  RightPortType=output  PseudoPeriodic=off  Frequencies=[]  Unit=1  AffineConversion=off
  PS-Simulink Converter2 : nesl_utility/PS-Simulink Converter  PhysicalDomain=network_engine_domain  SubClassName=ps_output  LeftPortType=input  RightPortType=output  PseudoPeriodic=off  Frequencies=[]  Unit=rad/s  AffineConversion=off
  PS-Simulink Converter3 : nesl_utility/PS-Simulink Converter  PhysicalDomain=network_engine_domain  SubClassName=ps_output  LeftPortType=input  RightPortType=output  PseudoPeriodic=off  Frequencies=[]  Unit=rad/s  AffineConversion=off
  PS-Simulink Converter4 : nesl_utility/PS-Simulink Converter  PhysicalDomain=network_engine_domain  SubClassName=ps_output  LeftPortType=input  RightPortType=output  PseudoPeriodic=off  Frequencies=[]  Unit=rad/s  AffineConversion=off
  Sensor Place : sm_lib/Frames and Transforms/Rigid Transform  TranslationMethod=Cartesian  TranslationStandardOffset=0  TranslationLengthUnit=m  TranslationStandardAxis=+Z  TranslationCartesianOffset=AARIAMAN.L(nL).S(nS).pose_p  TranslationROffset=0  TranslationROffsetUnits=m  TranslationZOffset=0  TranslationZOffsetUnits=m  TranslationThetaOffset=0  TranslationThetaOffsetUnits=deg  RotationMethod=RotationMatrix  RotationAngleUnits=deg  RotationStandardAxis=+Z  RotationAngle=0.0  RotationArbitraryAxis=[0 0 1]  FollAlignAxisA=+X  BaseAlignAxisA=+Y  FollAlignAxisB=+Y  BaseAlignAxisB=+Z  RotationSequenceAxes=FollowerAxes  RotationSequence=XYX  RotationSequenceAngles=[0 0 0]  RotationSequenceAnglesUnits=deg  RotationMatrix=AARIAMAN.L(nL).S(nS).pose_r
  Sum : Sum  Inputs=|++
  Sum1 : Sum  Inputs=|++
  Sum2 : Sum  Inputs=++|
  Transform Sensor : sm_lib/Frames and Transforms/Transform Sensor  MeasurementFrame=Follower  SenseAngle=off  SenseAxis=off  SenseAngle1=off  SenseAngle2=off  SenseAngle3=off  SenseQ=off  SenseR=on  SenseOmegaX=on  SenseOmegaY=on  SenseOmegaZ=on  SenseOmega1=off  SenseOmega2=off  SenseOmega3=off  SenseQDot=off  SenseRDot=off  SenseAlphaX=off  SenseAlphaY=off  SenseAlphaZ=off  SenseAlpha1=off  SenseAlpha2=off  SenseAlpha3=off  SenseQDDot=off  SenseRDDot=off  SenseX=on  SenseY=on  SenseZ=on  SenseRad=off  SenseAzim=off  SenseDist=off  SenseInc=off  SenseXDot=off  SenseYDot=off  SenseZDot=off  SenseRadDot=off  SenseAzimDot=off  SenseDistDot=off  SenseIncDot=off  SenseXDDot=on  SenseYDDot=on  SenseZDDot=on  SenseRadDDot=off  SenseAzimDDot=off  SenseDistDDot=off  SenseIncDDot=off
  a_noise : Subsystem
  coord_sens : sm_lib/Body Elements/Graphic  GraphicType=Marker  MarkerShape=Frame  MarkerSize=AARIAMAN.vis.coord_sizeS  GraphicVisPropType=SimpleVisualProperties  GraphicDiffuseColor=AARIAMAN.vis.col_s  GraphicSpecularColor=[0.5 0.5 0.5 1.0]  GraphicAmbientColor=[0.15 0.15 0.15 1.0]  GraphicEmissiveColor=[0.0 0.0 0.0 1.0]  GraphicShininess=75  GraphicOpacity=AARIAMAN.vis.opacity_s
      settings: SourceProductName=Simscape Multibody
  omega_noise : Subsystem
  Body Frame : PMIOPort  Port=1  Side=Left
  Reference Frame : PMIOPort  Port=2  Side=Left
  Out5 : Outport
  Out4 : Outport  Port=2
  Out2 : Outport  Port=3
  Out3 : Outport  Port=4
  wires:
  Sum2/1 -> Out5/1  "omega_measured"
  Sum/1 -> Sum1/1
  PS-Simulink Converter8/1 -> Gain3/1, Out3/1  "R_actual"
  Mux2/1 -> Gain1/1
  PS-Simulink Converter7/1 -> Mux1/3
  PS-Simulink Converter5/1 -> Mux1/1
  PS-Simulink Converter6/1 -> Mux1/2
  Mux/1 -> Gain/1
  PS-Simulink Converter4/1 -> Mux/3
  PS-Simulink Converter2/1 -> Mux/1
  PS-Simulink Converter3/1 -> Mux/2
  PS-Simulink Converter9/1 -> Mux2/1
  PS-Simulink Converter11/1 -> Mux2/3
  Mux1/1 -> Out2/1  "P_actual"
  PS-Simulink Converter10/1 -> Mux2/2
  Sum1/1 -> Out4/1  "a_measured"
  Gain3/1 -> Sum/2  "a_measured"
  omega_noise/1(noise) -> Sum2/1
  a_noise/1(noise) -> Sum1/2
  Gain/1 -> Sum2/2
  Gain1/1 -> Sum/1
  connections:
  Transform Sensor/RConn7 -- PS-Simulink Converter6/LConn1
  Transform Sensor/RConn8 -- PS-Simulink Converter7/LConn1
  PS-Simulink Converter8/LConn1 -- Transform Sensor/RConn2
  Transform Sensor/RConn6 -- PS-Simulink Converter5/LConn1
  Transform Sensor/RConn10 -- PS-Simulink Converter10/LConn1
  Transform Sensor/RConn5 -- PS-Simulink Converter4/LConn1
  Transform Sensor/LConn1 -- Reference Frame/RConn1
  Transform Sensor/RConn4 -- PS-Simulink Converter3/LConn1
  Transform Sensor/RConn9 -- PS-Simulink Converter9/LConn1
  Transform Sensor/RConn3 -- PS-Simulink Converter2/LConn1
  Sensor Place/LConn1 -- Body Frame/RConn1
  Transform Sensor/RConn11 -- PS-Simulink Converter11/LConn1
  Transform Sensor/RConn1 -- coord_sens/RConn1 -- Sensor Place/RConn1
